simulink model "mycfunc"  (R2017a)
settings: Solver=FixedStepAuto  StartTime=0.0  StopTime=10.0  RelTol=1e-3
settings Model: Creator=TSu  LastModifiedBy=TSu
settings SolverCC: AutoInsertRateTranBlk=on
settings RTWCC: Toolchain=MinGW64 v4.x | gmake (64-bit Windows)  BuildConfiguration=Specify

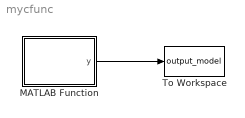
== system mycfunc ==
  MATLAB Function : MATLAB Function  TreatAsAtomicUnit=on
  To Workspace : ToWorkspace  VariableName=output_model  SaveFormat=Timeseries  SampleTime=-1
  wires:
  MATLAB Function/1(y) -> To Workspace/1

== matlab function mycfunc/MATLAB Function ==
  data: y output
function y = myfunc()

%#codegen
y = 21;
coder.cinclude('myMult2.h');
y = coder.ceval('myMult2', y);
% Specify the locations of myMult2.h and myMult2.c
coder.extrinsic('pwd', 'fullfile');
customDir = coder.const(fullfile(pwd, 'mycfiles'));
coder.updateBuildInfo('addIncludePaths', customDir);
coder.updateBuildInfo('addSourcePaths', customDir);
coder.updateBuildInfo('addSourceFiles', 'myMult2.c');
end
